simulink model "assignmenttorques"  (R2021b)
settings: Solver=VariableStepAuto  StartTime=0.0  StopTime=10  MaxStep=0.02  RelTol=1e-3
settings Model: Creator=emil1  LastModifiedBy=emil1

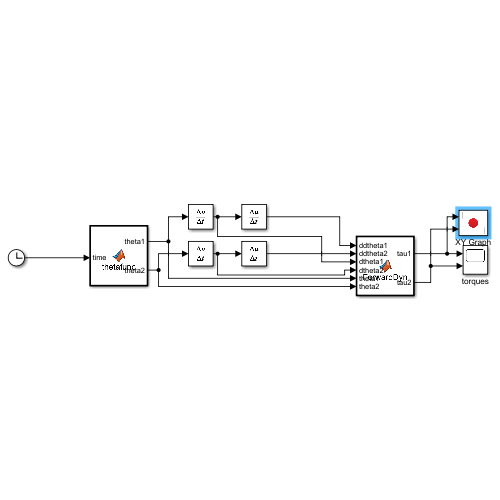
[thumbnail: Simulink's stored preview of the top-level diagram]
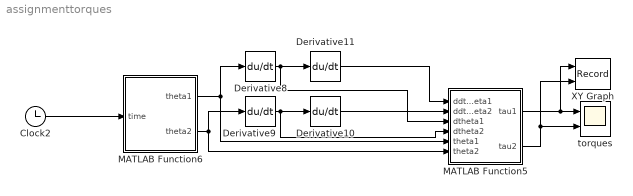
== system assignmenttorques ==
  Clock2 : Clock
  Derivative{8..11} (4 alike) : Derivative
  MATLAB Function5 : MATLAB Function  TreatAsAtomicUnit=on
  MATLAB Function6 : MATLAB Function  TreatAsAtomicUnit=on
  XY Graph : Record  FileSettingsInternal="{\"entries\":[{\"content\":{\"excelSettings\":{\"content\":{},\"type\":\"Streamout.ExcelSettings\"}},\"type\":\"Streamout.FileSettingStorage\",\"uuid\":\"a74af9a5-1507-42aa-ab8c-3dd4bc0be643\"}],\"packageUris\":[\"http://schema.mathworks.com/mf0/streamout_blocks/R2020a\"],\"version\":\"1.0\"}"  Layout=[1 1]  SignalsInternal="{\"entries\":[{\"content\":{\"signals\":[{\"content\":{\"blockPath\":[\"untitled/XY Graph\"],\"channel\":[],\"dimensions\":[1],\"domain\":\"untitled/XY Graph\",\"lineColor\":\"#a2142f\",\"plots\":[1],\"port\":1,\"sid\":[\"\"],\"signalID\":1214,\"signalName\":\"MATLAB Function5:1\"},\"type\":\"RecordBlkView.Signal\",\"uuid\":\"503ac62c-56bf-4f92-80a9-4ce138b2450b\"},{\"content\":{\"blockPath\":[\"untitled/XY Graph\"],\"channel\":[],\"dimensions\":[1],\"domain\":\"untitled/XY Graph\",\"lineColor\":\"#139fff\",\"plots\":[1],\"port\":2,\"sid\":[\"\"],\"signalID\":1218,\"signalName\":\"MATLAB Function5:2\"},\"type\":\"RecordBlkView.Signal\",\"uuid\":\"9910f31d-2ca0-4be1-a9b8-cb7478082b20\"}]},\"type\":\"RecordBlkView.InputSignals\",\"uuid\":\"20dba771-2f1b-478e-86e6-530756e8ea1e\"}],\"packageUris\":[\"http://schema.mathworks.com/mf0/streamout_blocks/R2020a\"],\"version\":\"1.0\"}"  VisualizationBindings="{\"xyplotplugin\":{\"info\":[{\"series\":[{\"bindingParametersList\":[{\"parameter\":\"X-Axis\",\"signalID\":1214,\"signalName\":\"MATLAB Function5:1\"},{\"parameter\":\"Y-Axis\",\"signalID\":1218,\"signalName\":\"MATLAB Function5:2\"}],\"seriesID\":53843}],\"subplotID\":1}]}}"  CompatibilityTag=XY
  torques : Scope  NumInputPorts=2
  wires:
  Derivative10/1 -> MATLAB Function5/2(ddtheta2)
  MATLAB Function5/1(tau1) -> XY Graph/1, torques/1
  Clock2/1 -> MATLAB Function6/1(time)
  MATLAB Function6/1(theta1) -> Derivative8/1, MATLAB Function5/5(theta1)
  MATLAB Function6/2(theta2) -> Derivative9/1, MATLAB Function5/6(theta2)
  Derivative9/1 -> Derivative10/1, MATLAB Function5/4(dtheta2)
  Derivative11/1 -> MATLAB Function5/1(ddtheta1)
  Derivative8/1 -> Derivative11/1, MATLAB Function5/3(dtheta1)
  MATLAB Function5/2(tau2) -> torques/2, XY Graph/2

== matlab function assignmenttorques/MATLAB Function5 ==
  data: ddtheta1 input; tau1 output; tau2 output; ddtheta2 input; dtheta1 input; dtheta2 input; theta1 input; theta2 input
function [tau1, tau2]= ForwardDyn(ddtheta1 ,ddtheta2, dtheta1, dtheta2, theta1, theta2)

g = 9.81;
p = 7806;
l1 = 1;
lc1 = l1/2; %mas siger
l2 = 0.5;
lc2 = l2/2;
m1 = 0.05*0.05*l1*p; 
m2 = 0.05*0.05*l2*p;
I1 = m1*l1*l1/3;
I2 = m2*l2*l2/12;
H11 = m1*lc1*lc1 + I1 + I2 + m2*(l1*l1 + lc2*lc2+2*l1*lc2*cos(theta2));
H22 = m1*lc2*lc2 + I2 ;
H12 = m2*(lc2*lc2 + 2*l1*lc2*cos(theta2)) + I2;
h = m2*l1*lc2*sin(theta2);
G1 = m1*g*lc1*cos(theta1) + m2*g*(l1*cos(theta1)+lc2*cos(theta1 + theta2));
G2 = m2*g*lc2*cos(theta1 + theta2); 
% tau

% H(theta)
M = [H11 H12;
     H12 H22];
%V ( theta dtheta)
V = [-h*dtheta2*dtheta2 - 2*h*dtheta1*dtheta2;
    h*dtheta1*dtheta1];
% G( theta )
G = [G1;G2];

ddtheta = [ddtheta1;ddtheta2];
tau = M*ddtheta + V + G;
tau1 = tau(1);
tau2 = tau(2);

== matlab function assignmenttorques/MATLAB Function6 ==
  data: time input; theta1 output; theta2 output
function [theta1, theta2]= thetafunc(time)

radian = pi*45/180;

theta1= 3*sin(pi*time);

theta2=0.5 * sin(3*pi*time+radian);
